simulink model "sim_punto_7"  (R2021b)
settings: Solver=VariableStepAuto  StartTime=0.0  StopTime=50  RelTol=1e-3
values from neighbouring files (symbols this model uses):
  A = [0 1 0 0 0 0 0 0 0 0 0 0 ... (first row only)    [punto7.m]
  A1 = [0 1 0 0 0 0 0 0 0 0 0 0 ... (first row only)    [punto7.m]
  B = [0; 0; 0; 0; 0; 0; 0; 0; 0; 0; 0; 1]    [punto7.m]
  C = [1 0 0 0 0 0 0 0 0 0 0 0]    [punto7.m]
  C_states = eye(12)    [punto7.m]
  D_states = [0 0 0 0 0 0 0 0 0 0 0 0]'    [punto7.m]
  N = 10    [punto7.m]
  N3 = 27    [punto7.m]
  Q = [1+q 0 0 0 0 0 0 0 0 0 0 0 ... (first row only)    [punto7.m]
  Qprimo = eye(13)    [punto7.m]
  R = 1    [punto7.m]
  S = [0 0 0 0 0 0 0 0 0 0 0 0 0 ... (first row only)    [punto7.m]
  Ts = 0.1    [punto7.m]
  Ubar = inv(g)*Ybar    [punto7.m]
  umax = 15    [punto7.m]
  umin = -15    [punto7.m]
  x0 = [0 0 0 0 0 0 0 0 0 0 0 0]'    [punto7.m]
  Xbar = -inv(A) * B * Ubar    [punto7.m]
  xmax = [repmat(xmax,N,1)]    [mympc_constraints.m]    (also in punto7.m = [10 inf 10 inf 10 inf 10 inf 10 inf 10 inf]')
  xmin = [repmat(xmin,N,1)]    [mympc_constraints.m]    (also in punto7.m = [-10 -inf -10 -inf -10 -inf -10 -inf -10 -inf -10 -inf]')
  Ybar = 1    [punto7.m]
undefined symbols (not defined in the file or in its folder): B1, mympc_constraints, mympc_velocityform, Sprimo
settings Model: Creator=danie  LastModifiedBy=danie

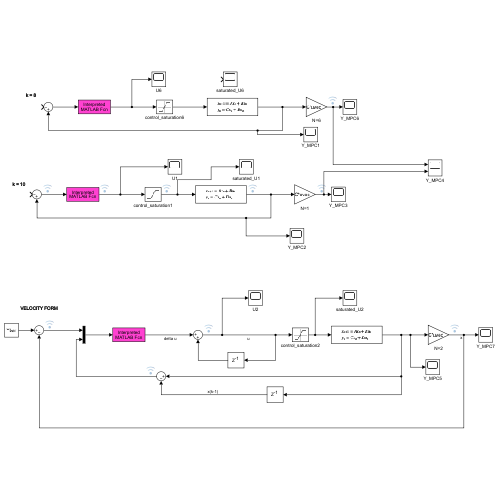
[thumbnail: Simulink's stored preview of the top-level diagram]
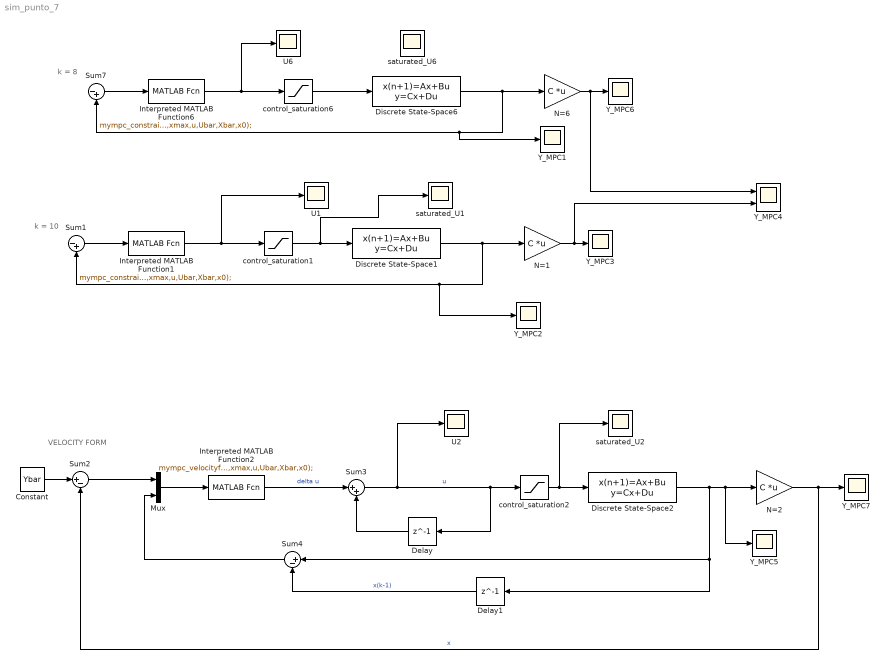
== system sim_punto_7 ==
  note: k = 8
  note: k = 10
  note: VELOCITY FORM
  Constant : Constant  Value=Ybar
  Delay : Delay  DelayLength=1
  Delay1 : Delay  DelayLength=1
  Discrete State-Space1 : DiscreteStateSpace  A=A  B=B  C=C_states  D=D_states  InitialCondition=x0  SampleTime=Ts
  Discrete State-Space2 : DiscreteStateSpace  A=A1  B=B1  C=C_states  D=D_states  InitialCondition=x0  SampleTime=Ts
  Discrete State-Space6 : DiscreteStateSpace  A=A1  B=B  C=C_states  D=D_states  InitialCondition=x0  SampleTime=Ts
  Interpreted MATLAB Function1 : MATLABFcn  MATLABFcn=mympc_constraints(A,B,Q,R,S,N3,umin,umax,xmin,xmax,u,Ubar,Xbar,x0);  OutputDimensions=1
  Interpreted MATLAB Function2 : MATLABFcn  MATLABFcn=mympc_velocityform(A,B,C,Qprimo,R,Sprimo,N,umin,umax,xmin,xmax,u,Ubar,Xbar,x0);  OutputDimensions=1  Output1D=off
  Interpreted MATLAB Function6 : MATLABFcn  MATLABFcn=mympc_constraints(A,B,Q,R,S,N3,umin,umax,xmin,xmax,u,Ubar,Xbar,x0);  OutputDimensions=1
  Mux : Mux  Inputs=2
  N=1 : Gain  Gain=C  Multiplication=Matrix(K*u) (u vector)
  N=2 : Gain  Gain=C  Multiplication=Matrix(K*u) (u vector)
  N=6 : Gain  Gain=C  Multiplication=Matrix(K*u) (u vector)
  Sum1 : Sum  Inputs=|-+
  Sum2 : Sum  Inputs=|+-
  Sum3 : Sum  Inputs=|++
  Sum4 : Sum  Inputs=|+-
  Sum7 : Sum  Inputs=|-+
  U1 : Scope
  U2 : Scope
  U6 : Scope
  Y_MPC{1..3,5..7} (6 alike) : Scope
  Y_MPC4 : Scope  NumInputPorts=2
  control_saturation1 : Saturate  UpperLimit=inf  LowerLimit=-inf
  control_saturation2 : Saturate  UpperLimit=inf  LowerLimit=-inf
  control_saturation6 : Saturate  UpperLimit=inf  LowerLimit=-inf
  saturated_U1 : Scope
  saturated_U2 : Scope
  saturated_U6 : Scope
  wires:
  Discrete State-Space6/1 -> Y_MPC1/1, Sum7/2, N=6/1
  N=6/1 -> Y_MPC4/1, Y_MPC6/1
  Sum7/1 -> Interpreted MATLAB Function6/1
  Interpreted MATLAB Function6/1 -> control_saturation6/1, U6/1
  control_saturation6/1 -> Discrete State-Space6/1
  Discrete State-Space1/1 -> Y_MPC2/1, Sum1/2, N=1/1
  N=1/1 -> Y_MPC4/2, Y_MPC3/1
  Sum1/1 -> Interpreted MATLAB Function1/1
  Interpreted MATLAB Function1/1 -> control_saturation1/1, U1/1
  control_saturation1/1 -> saturated_U1/1, Discrete State-Space1/1
  Discrete State-Space2/1 -> Delay1/1, Sum4/1, N=2/1, Y_MPC5/1
  N=2/1 -> Sum2/2, Y_MPC7/1  "x"
  Mux/1 -> Interpreted MATLAB Function2/1
  Constant/1 -> Sum2/1
  Interpreted MATLAB Function2/1 -> Sum3/1  "delta u"
  Delay/1 -> Sum3/2
  control_saturation2/1 -> saturated_U2/1, Discrete State-Space2/1
  Sum3/1 -> U2/1, Delay/1, control_saturation2/1  "u"
  Sum4/1 -> Mux/2
  Delay1/1 -> Sum4/2  "x(k-1)"
  Sum2/1 -> Mux/1
